simulink model "openLoopSimulation"  (R2024a)
settings: Solver=ode45  StartTime=0.0  StopTime=2000  RelTol=1e-3
undefined symbols (not defined in the file or in its folder): init, sat
libraries: sharedtransform x1, simulink_extras x1
settings Model: Creator=b_ant  LastModifiedBy=b_ant

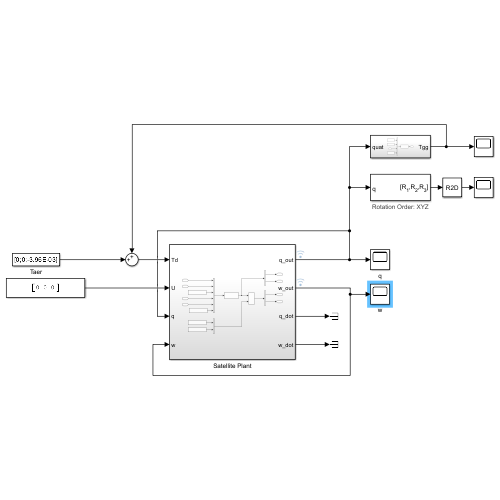
[thumbnail: Simulink's stored preview of the top-level diagram]
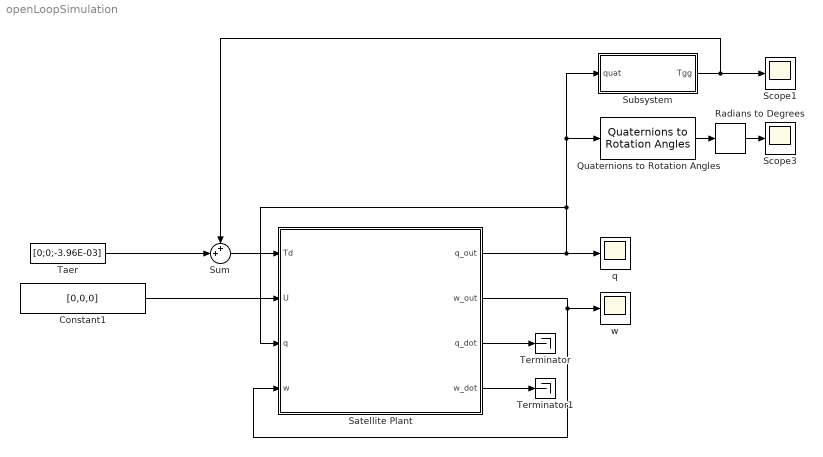
== system openLoopSimulation ==
  Constant1 : Constant  Value=[0,0,0]
  Quaternions to Rotation Angles : sharedtransform/Quaternions to Rotation Angles  rotationOrder=XYZ  aMode=aMode
  Radians to Degrees : simulink_extras/Transformations/Radians to Degrees
  Satellite Plant : Subsystem
  Scope1 : Scope
  Scope3 : Scope
  Subsystem : Subsystem
  Sum : Sum  Inputs=++|
  Taer : Constant  Value=[0;0;-3.96E-03]
  Terminator : Terminator
  Terminator1 : Terminator
  q : Scope
  w : Scope
  wires:
  Satellite Plant/2(w_out) -> w/1, Satellite Plant/4(w)
  Satellite Plant/3(q_dot) -> Terminator/1
  Satellite Plant/4(w_dot) -> Terminator1/1
  Quaternions to Rotation Angles/1 -> Radians to Degrees/1
  Radians to Degrees/1 -> Scope3/1
  Constant1/1 -> Satellite Plant/2(U)
  Satellite Plant/1(q_out) -> Subsystem/1(quat), Quaternions to Rotation Angles/1, Satellite Plant/3(q), q/1
  Subsystem/1(Tgg) -> Sum/1, Scope1/1
  Sum/1 -> Satellite Plant/1(Td)
  Taer/1 -> Sum/2

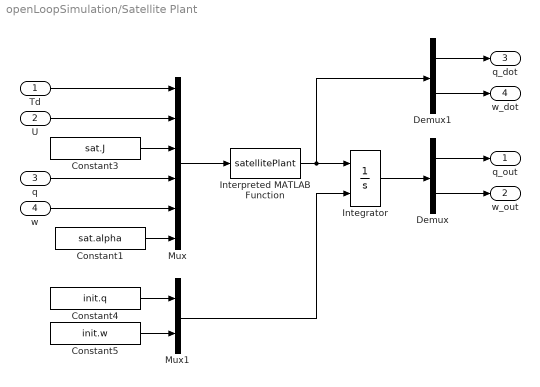
== system openLoopSimulation/Satellite Plant ==
  Td : Inport
  U : Inport  Port=2
  q : Inport  Port=3
  w : Inport  Port=4
  Constant1 : Constant  Value=sat.alpha
  Constant3 : Constant  Value=sat.J
  Constant4 : Constant  Value=init.q
  Constant5 : Constant  Value=init.w
  Demux : Demux  Outputs=2
  Demux1 : Demux  Outputs=2
  Integrator : Integrator  InitialConditionSource=external
  Interpreted MATLAB Function : MATLABFcn  MATLABFcn=satellitePlant
  Mux : Mux  Inputs=6
  Mux1 : Mux  Inputs=2
  q_out : Outport
  w_out : Outport  Port=2
  q_dot : Outport  Port=3
  w_dot : Outport  Port=4
  wires:
  Td/1 -> Mux/1
  Mux/1 -> Interpreted MATLAB Function/1
  U/1 -> Mux/2
  Interpreted MATLAB Function/1 -> Demux1/1, Integrator/1
  Constant5/1 -> Mux1/2
  Constant4/1 -> Mux1/1
  Mux1/1 -> Integrator/2
  Integrator/1 -> Demux/1
  Demux/1 -> q_out/1
  Demux/2 -> w_out/1
  Demux1/1 -> q_dot/1
  Demux1/2 -> w_dot/1
  Constant3/1 -> Mux/3
  q/1 -> Mux/4
  w/1 -> Mux/5
  Constant1/1 -> Mux/6

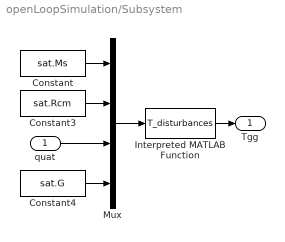
== system openLoopSimulation/Subsystem ==
  quat : Inport
  Constant : Constant  Value=sat.Ms
  Constant3 : Constant  Value=sat.Rcm
  Constant4 : Constant  Value=sat.G
  Interpreted MATLAB Function : MATLABFcn  MATLABFcn=T_disturbances
  Mux : Mux
  Tgg : Outport
  wires:
  Constant/1 -> Mux/1
  Constant3/1 -> Mux/2
  Mux/1 -> Interpreted MATLAB Function/1
  quat/1 -> Mux/3
  Constant4/1 -> Mux/4
  Interpreted MATLAB Function/1 -> Tgg/1
